simulink model "Motor_Scheme"  (R2021b)
settings: Solver=FixedStepAuto  StartTime=0.0  StopTime=inf  FixedStep=Ts  RelTol=1e-3  EnableMultiTasking=on
undefined symbols (not defined in the file): Ts
libraries: mbedblockslib x3, stm_qeplib x1
settings Model: SILPILSystemUnderTest=refmodels  ExtModeTrigDuration=10  Creator=Luigi  LastModifiedBy=UTENTE
settings DataIOCC: DSMLogging=off  ReturnWorkspaceOutputs=off
settings OptimizationCC: BlockReduction=off  ConditionallyExecuteInputs=off  EnhancedBackFolding=on  PassReuseOutputArgsAs=Individual arguments  ZeroExternalMemoryAtStartup=off  ZeroInternalMemoryAtStartup=off  MaxStackSize=64  AccelVerboseBuild=on  OptimizeBlockOrder=speed  DifferentSizesBufferReuse=on  OptimizationCustomize=off  EfficientTunableParamExpr=on
settings DebuggingCC: ParameterTunabilityLossMsg=error
settings HardwareCC: ProdBitPerPointer=32  ProdBitPerSizeT=32  ProdBitPerPtrDiffT=32  ProdLargestAtomicInteger=Long  ProdLargestAtomicFloat=Double  ProdWordSize=32  ProdLongLongMode=on  ProdHWDeviceType=ARM Compatible->ARM Cortex
settings SFSimCC: SFSimEcho=off  EnableRuntimeRecursion=off  MATLABDynamicMemAlloc=off
settings RTWCC: Description=Embedded Coder  SystemTargetFile=ert.tlc  HardwareBoard=STM32 Nucleo F401RE  TemplateMakefile=ert_default_tmf  GenerateReport=on  Toolchain=GNU Tools for ARM Embedded Processors  IncludeHyperlinkInReport=on  PortableWordSizes=on  CodeExecutionProfiling=on  CodeProfilingInstrumentation=coarse
settings CodeAppCC: ForceParamTrailComments=on  IgnoreCustomStorageClasses=off  OperatorAnnotations=on  SimulinkDataObjDesc=on  SFDataObjDesc=on  InsertBlockDesc=on
settings ERTTargetCC: ExtModeTransport=3  ExtModeStaticAlloc=on  ExtModeStaticAllocSize=2000  ExtModeMexFile=ext_xcp  ExtModeIntrfLevel=Level2 - Open

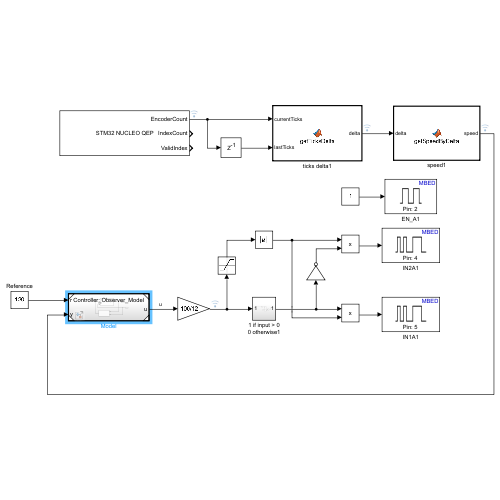
[thumbnail: Simulink's stored preview of the top-level diagram]
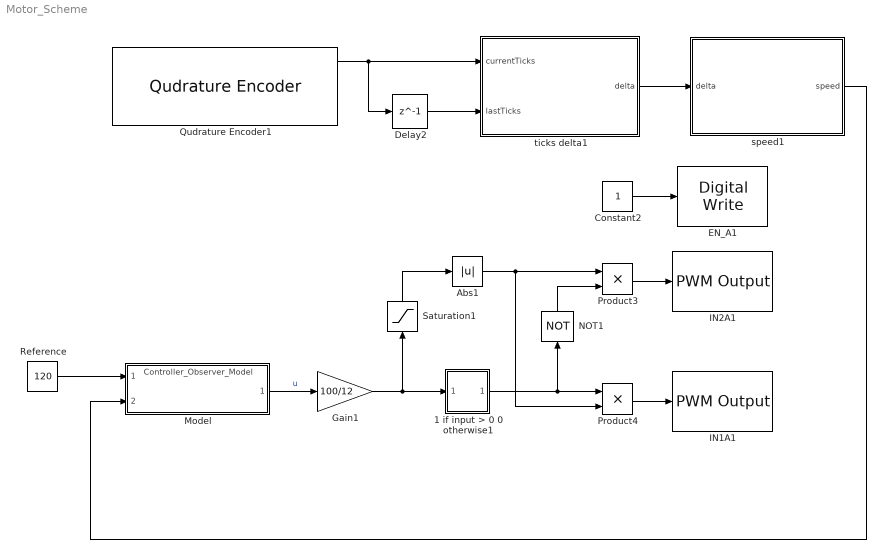
== system Motor_Scheme ==
  1 if input > 0 0 otherwise1 : Subsystem
  Abs1 : Abs
  Constant2 : Constant
  Delay2 : Delay  DelayLength=1  InitialCondition=0
  EN_A1 : mbedblockslib/Digital Write  Pin=2  Direction=output
      settings: SourceProductBaseCode=MICROBIT,NUCLEO,STMICRODIS
  Gain1 : Gain  Gain=100/12
  IN1A1 : mbedblockslib/PWM Output  Pin=5  EnableInputFrequency=off  InitialFrequency=pwmFreq  InitialDutyCycle=0  NotificationType=None
      settings: SourceProductBaseCode=MICROBIT,NUCLEO,STMICRODIS
  IN2A1 : mbedblockslib/PWM Output  Pin=4  EnableInputFrequency=off  InitialFrequency=pwmFreq  InitialDutyCycle=0  NotificationType=None
      settings: SourceProductBaseCode=MICROBIT,NUCLEO,STMICRODIS
  Model : ModelReference  ModelNameDialog=Controller_Observer_Model.slx  SimulationMode=Normal  ModelReferenceVersion=1.2
  NOT1 : Logic  Operator=NOT  IconShape=distinctive  AllPortsSameDT=off  OutDataTypeStr=boolean
  Product3 : Product
  Product4 : Product
  Qudrature Encoder1 : stm_qeplib/Qudrature Encoder  SampleTime=Ts
  Reference : Constant  Value=120
  Saturation1 : Saturate  UpperLimit=100  LowerLimit=-100
  speed1 : MATLAB Function  TreatAsAtomicUnit=on
  ticks delta1 : MATLAB Function  TreatAsAtomicUnit=on
  wires:
  Reference/1 -> Model/1
  Model/1 -> Gain1/1  "u"
  Qudrature Encoder1/1 -> ticks delta1/1(currentTicks), Delay2/1
  Saturation1/1 -> Abs1/1
  Product3/1 -> IN2A1/1
  Constant2/1 -> EN_A1/1
  Delay2/1 -> ticks delta1/2(lastTicks)
  NOT1/1 -> Product3/2
  Gain1/1 -> Saturation1/1, 1 if input > 0 0 otherwise1/1(In1)
  Abs1/1 -> Product4/2, Product3/1
  ticks delta1/1(delta) -> speed1/1(delta)
  Product4/1 -> IN1A1/1
  speed1/1(speed) -> Model/2
  1 if input > 0 0 otherwise1/1(Out1) -> Product4/1, NOT1/1

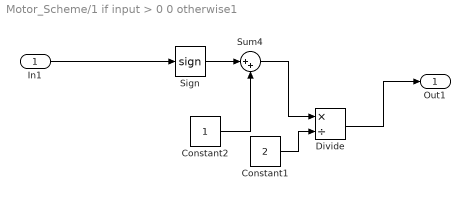
== system Motor_Scheme/1 if input > 0 0 otherwise1 ==
  In1 : Inport
  Constant1 : Constant  Value=2
  Constant2 : Constant
  Divide : Product  Inputs=*/
  Sign : Signum
  Sum4 : Sum  Inputs=|++
  Out1 : Outport
  wires:
  Sum4/1 -> Divide/1
  Constant2/1 -> Sum4/2
  Sign/1 -> Sum4/1
  Divide/1 -> Out1/1
  In1/1 -> Sign/1
  Constant1/1 -> Divide/2

== matlab function Motor_Scheme/ticks delta1 ==
  data: currentTicks input; delta output; lastTicks input; Ts parameter
function delta = getTicksDelta(currentTicks,lastTicks,Ts)

currentTicks = double(currentTicks);
lastTicks = double(lastTicks);

if abs(currentTicks-lastTicks) <= ceil(8400*Ts) 
	 delta = currentTicks-lastTicks;
else
if lastTicks>currentTicks
	 delta = currentTicks+2^16-1-lastTicks;
else
	 delta = currentTicks-2^16+1-lastTicks;
	end
end

end

== matlab function Motor_Scheme/speed1 ==
  data: delta input; speed output; Ts parameter
function speed = getSpeedByDelta(delta,Ts)

speed = delta*60/(3591.84*Ts);

end
